simulink model "PWM_emulator"  (R2016a)
settings: Solver=FixedStepDiscrete  StartTime=0.0  StopTime=0.02  FixedStep=Tsim  RelTol=1e-3
values from neighbouring files (symbols this model uses):
  Tosc = 1/Fosc    (= 1.49011611938e-08)    [PWM_params.m]
settings Model: SimulationMode=accelerator  Creator=Cosmin  LastModifiedBy=Cosmin

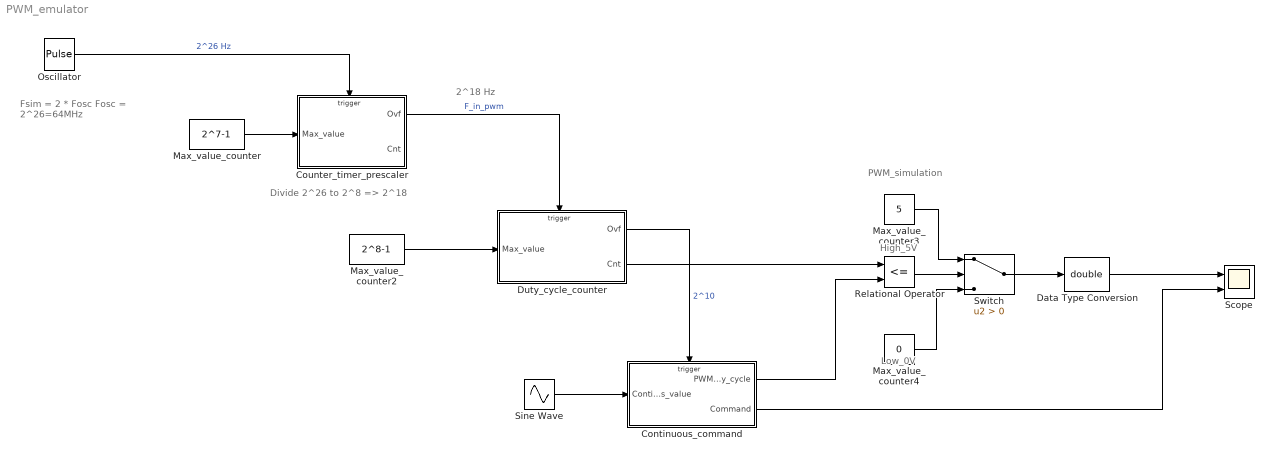
== system PWM_emulator ==
  note: PWM_simulation
  note: 2^18 Hz
  note: Divide 2^26 to 2^8 => 2^18
  note: Fsim = 2 * Fosc
      | Fosc = 2^26=64MHz
  note: High_5V
  note: Low_0V
  Continuous_command : Subsystem
  Counter_timer_prescaler : Subsystem
  Data Type Conversion : DataTypeConversion  OutDataTypeStr=double
  Duty_cycle_counter : Subsystem
  Max_value_counter : Constant  Value=2^7-1  OutDataTypeStr=uint16
  Max_value_counter2 : Constant  Value=2^8-1  OutDataTypeStr=uint16
  Max_value_counter3 : Constant  Value=5  OutDataTypeStr=uint16
  Max_value_counter4 : Constant  Value=0  OutDataTypeStr=uint16
  Oscillator : DiscretePulseGenerator  PulseType=Time based  Period=Tosc  PulseWidth=50
  Relational Operator : RelationalOperator  Operator=<=  OutDataTypeStr=boolean
  Scope : Scope  NumInputPorts=2
  Sine Wave : Sin  Amplitude=5  Frequency=20*pi
  Switch : Switch  Criteria=u2 > Threshold
  wires:
  Oscillator/1 -> Counter_timer_prescaler/Trigger  "2^26 Hz"
  Max_value_counter/1 -> Counter_timer_prescaler/1(Max_value)
  Counter_timer_prescaler/1(Ovf) -> Duty_cycle_counter/Trigger  "F_in_pwm"
  Max_value_counter2/1 -> Duty_cycle_counter/1(Max_value)
  Data Type Conversion/1 -> Scope/1
  Continuous_command/2(Command) -> Scope/2
  Duty_cycle_counter/1(Ovf) -> Continuous_command/Trigger  "2^10"
  Max_value_counter4/1 -> Switch/3
  Max_value_counter3/1 -> Switch/1
  Relational Operator/1 -> Switch/2
  Duty_cycle_counter/2(Cnt) -> Relational Operator/1
  Switch/1 -> Data Type Conversion/1
  Continuous_command/1(PWM_Duty_cycle) -> Relational Operator/2
  Sine Wave/1 -> Continuous_command/1(Continuous_value)

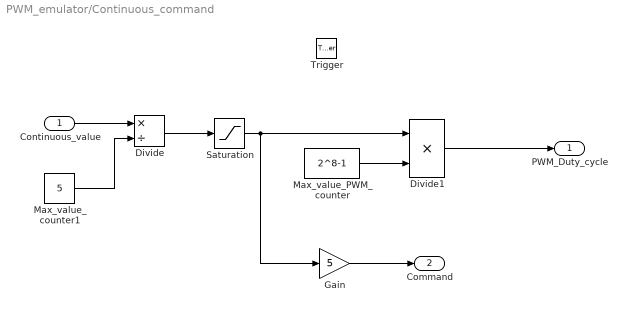
== system PWM_emulator/Continuous_command ==
  Continuous_value : Inport
  Trigger : TriggerPort  VariantControl=Variant  PortDimensions=1
  Divide : Product  Inputs=*/
  Divide1 : Product  Inputs=**  OutDataTypeStr=uint16
  Gain : Gain  Gain=5
  Max_value_PWM_counter : Constant  Value=2^8-1  OutDataTypeStr=uint16
  Max_value_counter1 : Constant  Value=5  OutDataTypeStr=uint16
  Saturation : Saturate  UpperLimit=1  LowerLimit=0
  PWM_Duty_cycle : Outport
  Command : Outport  Port=2
  wires:
  Max_value_PWM_counter/1 -> Divide1/2
  Divide1/1 -> PWM_Duty_cycle/1
  Divide/1 -> Saturation/1
  Max_value_counter1/1 -> Divide/2
  Saturation/1 -> Gain/1, Divide1/1
  Gain/1 -> Command/1
  Continuous_value/1 -> Divide/1

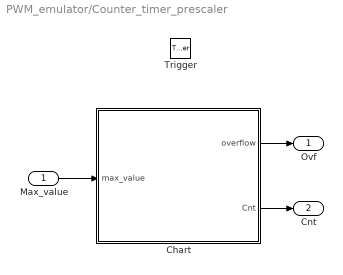
== system PWM_emulator/Counter_timer_prescaler ==
  Max_value : Inport
  Trigger : TriggerPort  VariantControl=Variant  PortDimensions=1
  Chart : Stateflow chart  TreatAsAtomicUnit=on
  Ovf : Outport  OutDataTypeStr=uint8
  Cnt : Outport  Port=2  OutDataTypeStr=uint16
  wires:
  Chart/1(overflow) -> Ovf/1
  Max_value/1 -> Chart/1(max_value)
  Chart/2(Cnt) -> Cnt/1

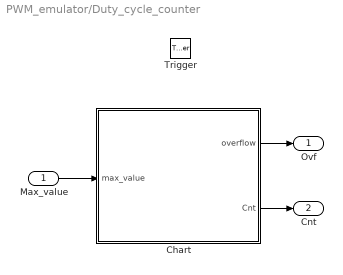
== system PWM_emulator/Duty_cycle_counter ==
  Max_value : Inport
  Trigger : TriggerPort  VariantControl=Variant  PortDimensions=1
  Chart : Stateflow chart  TreatAsAtomicUnit=on
  Ovf : Outport  OutDataTypeStr=uint8
  Cnt : Outport  Port=2  OutDataTypeStr=uint16
  wires:
  Chart/2(Cnt) -> Cnt/1
  Max_value/1 -> Chart/1(max_value)
  Chart/1(overflow) -> Ovf/1

== stateflow chart PWM_emulator/Duty_cycle_counter/Chart ==
  (default) -> (junction 1)
  (junction 1) -> (junction 3) : {count = count + 1;}
  (junction 3) -> (junction 5) [order 2] : {count=uint16(0);overflow=uint8(1);}
  (junction 3) -> (junction 5) [order 1] : [count<=max_value]{overflow=uint8(0);}
  (junction 5) -> (junction 11) : {Cnt=count;}
  data: max_value input uint16; overflow output uint8 =uint8(0); count local uint16 =uint16(0); Cnt output uint16 =uint16(0); data local

== stateflow chart PWM_emulator/Counter_timer_prescaler/Chart ==
  (default) -> (junction 1)
  (junction 1) -> (junction 3) : {count = count + 1;}
  (junction 3) -> (junction 5) [order 2] : {count=uint16(0);overflow=uint8(1);}
  (junction 3) -> (junction 5) [order 1] : [count<=max_value]{overflow=uint8(0);}
  (junction 5) -> (junction 11) : {Cnt=count;}
  data: max_value input uint16; overflow output uint8 =uint8(0); count local uint16 =uint16(0); Cnt output uint16 =uint16(0); data local
